simulink model "PR_Planar_Testbench_2018"  (R2024a)
settings: Solver=FixedStepDiscrete  StartTime=0.0  StopTime=inf  FixedStep=param.t_sample  RelTol=1e-3
undefined symbols (not defined in the file): max_qa, min_qa, param, slave3
libraries: Cust_Library_planarPKM x54, simulink_extras x27, dspswit3 x24, simulink x22, etherlab_lib x12
(part 1 of 6)
settings Model: SimulationMode=accelerator  ExtModeTrigDuration=10000  ExtModeArchiveMode=auto  ExtModeArchiveFileName=measurement_data  ExtModeArchiveDirName=/home/pkr_devpc/Schreibtisch/Git/3rrr_pkm/Versuchsstand/result  ExtModeLogAll=off  Creator=schappler  LastModifiedBy=mohammad_admin
settings SolverCC: AlgebraicLoopSolver=TrustRegion  MinimalZcImpactIntegration=on
settings DataIOCC: SaveOutput=off  SignalLogging=off  SaveTime=off  ReturnWorkspaceOutputs=off
settings OptimizationCC: BufferReuse=off  GlobalBufferReuse=off  ExpressionFolding=off  LocalBlockOutputs=off  OptimizeDataStoreBuffers=off  BusAssignmentInplaceUpdate=off
settings DebuggingCC: ReadBeforeWriteMsg=DisableAll  WriteAfterWriteMsg=DisableAll  WriteAfterReadMsg=DisableAll  MultiTaskDSMMsg=none  UnconnectedInputMsg=warning  UnconnectedOutputMsg=warning  UnconnectedLineMsg=warning  ArithmeticOperatorsInVariantConditions=warning
settings ModelReferenceCC: UpdateModelReferenceTargets=IfOutOfDate  EnableRefExpFcnMdlSchedulingChecks=on
settings SFSimCC: SFSimEcho=off  CustomCodeUndefinedFunction=UseInterfaceOnly
settings RTWCC: Description=EtherLab PREEMT_RT Real-Time Target  SystemTargetFile=etherlab.tlc  TemplateMakefile=etherlab_hrt.tmf  GenerateReport=on  LaunchReport=on  GPUComputeCapability=3.5
settings STFCustomTargetCC: UseToolchainInfoCompliant=off  SystemTargetFile=etherlab.tlc
settings GRTTargetCC: ParMdlRefBuildCompliant=off  CompOptLevelCompliant=off  ConcurrentExecutionCompliant=off  CombineOutputUpdateFcns=off  MatFileLogging=off  CPPClassGenCompliant=off  GRTInterface=on  UseToolchainInfoCompliant=off  ExtMode=on  ExtModeStaticAlloc=on  ExtModeStaticAllocSize=2000000000  ExtModeMexArgs='10.144.130.139' 0 17725  RTWCAPISignals=on  RTWCAPIParams=on

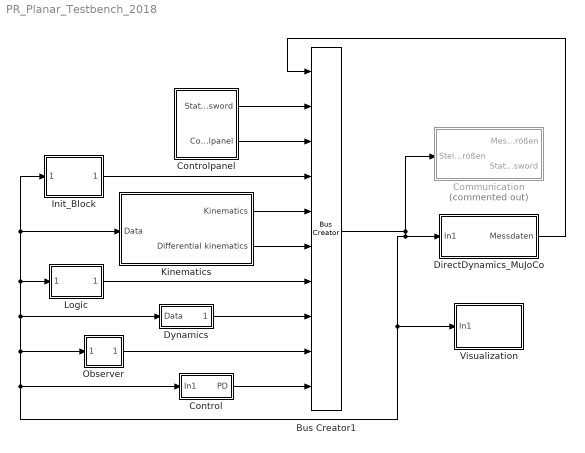
== system PR_Planar_Testbench_2018 ==
  Bus Creator1 : BusCreator  Inputs=10
  Communication : Subsystem  Commented=on
  Control : Subsystem
  Controlpanel : Subsystem
  DirectDynamics_MuJoCo : Subsystem
  Dynamics : Subsystem
  Init_Block : Subsystem
  Kinematics : Subsystem
  Logic : Subsystem
  Observer : Subsystem
  Visualization : Subsystem
  wires:
  Bus Creator1/1 -> Communication/1(Stellgrößen), Init_Block/1(Start_int), Kinematics/1(Data), Logic/1(Data), Dynamics/1(Data), Observer/1(In1), Control/1(In1), Visualization/1(In1), DirectDynamics_MuJoCo/1(In1)
  Control/1(PD) -> Bus Creator1/10
  Observer/1(Obs) -> Bus Creator1/9
  Dynamics/1(1) -> Bus Creator1/8
  Logic/1(Out1) -> Bus Creator1/7
  Kinematics/2(Differential kinematics) -> Bus Creator1/6
  Kinematics/1(Kinematics) -> Bus Creator1/5
  Init_Block/1(Out1) -> Bus Creator1/4
  Controlpanel/2(Controlpanel) -> Bus Creator1/3
  DirectDynamics_MuJoCo/1(Messdaten) -> Bus Creator1/1
  Controlpanel/1(Statusword) -> Bus Creator1/2

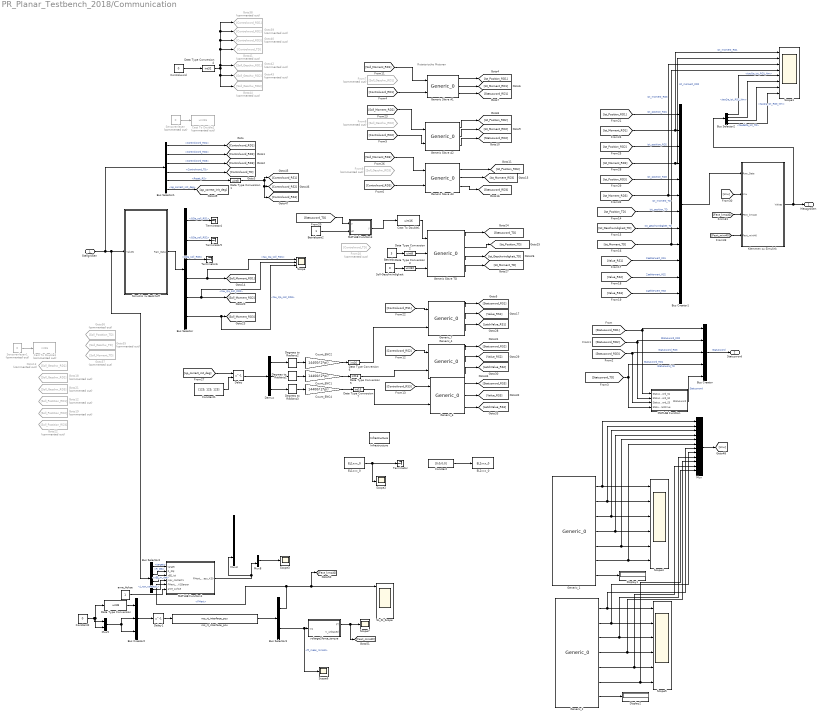
== system PR_Planar_Testbench_2018/Communication ==
  note: Rotatorische Motoren
  Stellgrößen : Inport
  Betriebsart : Constant  Value=3  SampleTime=-1
  Betriebsart2 : Constant  SampleTime=-1
  Bus Creator : BusCreator  Inputs=5
  Bus Creator1 : BusCreator  Inputs=12
  Bus Creator2 : BusCreator  Inputs=3
  Bus Selector : BusSelector  OutputSignals=QDa_soll_RD1,QDa_soll_RD2,QDa_soll_RD3,tau_Qa_soll_RD1,tau_Qa_soll_RD2,tau_Qa_soll_RD3
  Bus Selector1 : BusSelector  OutputSignals=State Variables.Controlword_RD1,State Variables.Controlword_RD2,State Variables.Controlword_RD3,State Variables.Controlword_TD,Controlpanel.Reset_RS,Kinematics_currentValues.qp_correct_init_deg
  Bus Selector2 : BusSelector  OutputSignals=tauQa_ist_RD1_Nm,tauQa_ist_RD2_Nm,tauQa_ist_RD3_Nm,taudelta_ist_TD
  Bus Selector3 : BusSelector  OutputSignals=FMext,ft_meas_mini40
  Bus Selector4 : BusSelector  OutputSignals=Controlpanel.target,Kontakt.R_0Gj,Kinematics_currentValues.xEE_m_rad,Kontakt.J_xpx_contact1
  Cast To Double1 : DataTypeConversion  OutDataTypeStr=uint16  SaturateOnIntegerOverflow=off  RndMeth=Floor
  Cast To Double2 : DataTypeConversion  Commented=on  OutDataTypeStr=uint16  SaturateOnIntegerOverflow=off  RndMeth=Floor
  Cast To Double3 : DataTypeConversion  Commented=on  OutDataTypeStr=int16  SaturateOnIntegerOverflow=off  RndMeth=Floor
  Constant : Constant  Value=[0;0;0;0]  SampleTime=param.t_sample
  Constant1 : Constant  Value=[123; 123; 123]  SampleTime=param.t_sample
  Constant2 : Constant  Value=0  SampleTime=-1
  "Controlword " : Constant  Value=0  SampleTime=-1
  Count_ENC1 : Gain  Gain=14400/(2*pi)  ParamDataTypeStr=double  OutDataTypeStr=double
  Count_ENC2 : Gain  Gain=14400/(2*pi)  ParamDataTypeStr=double  OutDataTypeStr=double
  Count_ENC4 : Gain  Gain=14400/(2*pi)  ParamDataTypeStr=double  OutDataTypeStr=double
  Data Type Conversion : DataTypeConversion  OutDataTypeStr=uint8  SaturateOnIntegerOverflow=off  RndMeth=Floor
  Data Type Conversion1 : DataTypeConversion  OutDataTypeStr=uint8  SaturateOnIntegerOverflow=off  RndMeth=Floor
  Data Type Conversion2 : DataTypeConversion  OutDataTypeStr=uint8  SaturateOnIntegerOverflow=off  RndMeth=Floor
  Data Type Conversion3 : DataTypeConversion  OutDataTypeStr=uint32  SaturateOnIntegerOverflow=off  RndMeth=Floor
  Data Type Conversion4 : DataTypeConversion  OutDataTypeStr=int32  SaturateOnIntegerOverflow=off  RndMeth=Floor
  Data Type Conversion5 : DataTypeConversion  OutDataTypeStr=int16  SaturateOnIntegerOverflow=off  RndMeth=Floor
  Data Type Conversion6 : DataTypeConversion  OutDataTypeStr=int16  SaturateOnIntegerOverflow=off  RndMeth=Floor
  Data Type Conversion7 : DataTypeConversion  OutDataTypeStr=int16  SaturateOnIntegerOverflow=off  RndMeth=Floor
  Degrees to Radians1 : simulink_extras/Transformations/Degrees to Radians
  Degrees to Radians2 : simulink_extras/Transformations/Degrees to Radians
  Degrees to Radians3 : simulink_extras/Transformations/Degrees to Radians
  Delay : Delay  DelayLength=1  InitialConditionSource=Input port  InitialCondition=[122;122;123]
      settings: InputPortMap=u0,p4
  Delay1 : Delay  DelayLength=1
  Demux : Demux  Outputs=3
  Display1 : Display
  Display2 : Display
  EL1xxx_0 : etherlab_lib/EtherCAT/Beckhoff/EL1xxx_0  master=0  index=6  model=EL1004  revision=[65810514 1048576]  vector=on  tsample=param.t_sample  debug=0
  EL2xxx_0 : etherlab_lib/EtherCAT/Beckhoff/EL2xxx_0  master=0  index=5  model=EL2004  revision=[131346514 1048576]  vector=on  diag=off  tsample=param.t_sample  debug=0
  From10 : From  Commented=on  GotoTag=Controlword_TD
  From7 : From  Commented=on  GotoTag=Soll_Geschw_RD1
  From8 : From  Commented=on  GotoTag=Soll_Geschw_RD2
  From9 : From  Commented=on  GotoTag=Soll_Geschw_RD3
  Generic Slave A1 : etherlab_lib/EtherCAT/Generic_0  master=0  index=1  rv=slave1_Stromregelung  param=[]  tsample=0.001  debug=0
  Generic Slave A2 : etherlab_lib/EtherCAT/Generic_0  master=0  index=2  rv=slave1_Stromregelung  param=[]  tsample=0.001  debug=0
  Generic Slave A3 : etherlab_lib/EtherCAT/Generic_0  master=0  index=0  rv=slave1_Stromregelung  param=[]  tsample=0.001  debug=0
  Generic Slave TD : etherlab_lib/EtherCAT/Generic_0  master=0  index=3  rv=slave3()  param=[]  tsample=0.001  debug=0
  Generic_1 : etherlab_lib/EtherCAT/Generic_0  master=0  index=10  rv=imu_etherlab_config  param=[]  tsample=1e-3  debug=0
  Generic_2 : etherlab_lib/EtherCAT/Generic_0  master=0  index=11  rv=imu_etherlab_config  param=[]  tsample=1e-3  debug=0
  Generic_4 : etherlab_lib/EtherCAT/Generic_0  master=0  index=9  rv=slave7  param=[]  tsample=0.001  debug=0
  Generic_6 : etherlab_lib/EtherCAT/Generic_0  master=0  index=7  rv=slave7  param=[]  tsample=0.001  debug=0
  Generic_7 : etherlab_lib/EtherCAT/Generic_0  master=0  index=8  rv=slave7  param=[]  tsample=0.001  debug=0
  Goto12 : Goto  Commented=on  GotoTag=Soll_Postition_RD1
  Goto13 : Goto  Commented=on  GotoTag=Soll_Geschw_RD1
  Goto18 : Goto  Commented=on  GotoTag=Soll_Geschw_RD2
  Goto19 : Goto  Commented=on  GotoTag=Soll_Postition_RD2
  Goto21 : Goto  Commented=on  GotoTag=Soll_Geschw_RD3
  Goto22 : Goto  Commented=on  GotoTag=Soll_Postition_RD3
  Goto35 : Goto  Commented=on  GotoTag=Soll_Geschw_TD
  Goto36 : Goto  Commented=on  GotoTag=Soll_Postition_TD
  Goto37 : Goto  Commented=on  GotoTag=Soll_Moment_TD
  Goto38 : Goto  Commented=on  GotoTag=Controlword_RD1
  Goto39 : Goto  Commented=on  GotoTag=Controlword_RD2
  Goto40 : Goto  Commented=on  GotoTag=Controlword_RD3
  Goto41 : Goto  Commented=on  GotoTag=Controlword_TD
  Goto42 : Goto  Commented=on  GotoTag=Soll_Geschw_RD1
  Goto43 : Goto  Commented=on  GotoTag=Soll_Geschw_RD2
  Goto44 : Goto  Commented=on  GotoTag=Soll_Geschw_RD3
  Infrastructure : etherlab_lib/EtherCAT/Beckhoff/Infrastructure  master=0  index=4  model=EK1100  revision=[72100946 0]  vector=off  tsample=param.t_sample  debug=0
  Klemmen zu Simulink : Subsystem
  MATLAB Function : MATLAB Function  TreatAsAtomicUnit=on
  MATLAB Function1 : MATLAB Function  TreatAsAtomicUnit=on
  MATLAB Function3 : MATLAB Function  TreatAsAtomicUnit=on
  Mux : Mux  Inputs=12
  Mux3 : Mux
  Mux5 : Mux  Inputs=2
  Mux8 : Mux  Inputs=2
  SL_IN_Scope : Scope  NumInputPorts=5
  Scope : Scope  NumInputPorts=3
  Scope1 : Scope  NumInputPorts=8
  Scope{2..3,6..7} (4 alike) : Scope
  Scope4 : Scope  NumInputPorts=6
  Scope5 : Scope  NumInputPorts=6
  Sensorenlesen : Constant  Commented=on  Value=0  SampleTime=-1
  Sensorenlesen1 : Constant  Commented=on  Value=0  SampleTime=-1
  Simulink zu Beckhoff : Subsystem
  Soll-Geschwindigkeit : Constant  Value=0  SampleTime=-1
  Terminator{,4..6} (4 alike) : Terminator
  anre_Achse : Constant  SampleTime=-1
  ros_rt_interface_pcu : S-Function  FunctionName=ros_rt_interface_pcu  SFunctionDeploymentMode=off  EnableBusSupport=off  mask(Legacy Function){SFunctionSpec=void SL_io_func(SL_OUT_type u1[1], SL_IN_type y1[1]), ShowSpec=on}
      mask prompts: ShowSpec "Display function specification"
      mask help:
      | This block allows you to call the legacy functions specified by the following Legacy Code Tool definition:
      | def.SFunctionName = 'ros_rt_interface_pcu';
      | def.OutputFcnSpec = 'void SL_io_func(SL_OUT_type u1[1], SL_IN_type y1[1])';
      | def.StartFcnSpec = 'void SL_start_func()';
      | def.TerminateFcnSpec = 'void SL_terminate_func()';
      | def.HeaderFiles = {'SL_func.h'};
      | def.SourceFiles = {'../ros_rt_interface/ros_rt_core/SL_func_dummy.cpp'};
      | def.TargetLibFiles = {'libros_sl_interface.so'};
      | def.IncPaths = {'../ros_rt_interface/ros_rt_core'};
      mask Help: <p>This block was generated automatically by the Legacy Code Tool. For detailed help on this tool, call<a href="matlab:legacy_code('help')"> legacy_code('help')</a>.</p>
      mask Callback ShowSpec:
      | if strcmp(get_param(gcbh, 'ShowSpec'), 'on')
      |   set_param(gcbh, 'MaskDisplay', sprintf('fprintf(''%s'');', get_param(gcbh, 'SFunctionSpec')));
      | else
      |   set_param(gcbh, 'MaskDisplay', sprintf('fprintf(''%s'');', get_param(gcbh, 'FunctionName')));
      | end
      mask Display: fprintf('void SL_io_func(SL_OUT_type u1[1], SL_IN_type y1[1])');
  voltage2force_torque : Subsystem
  Messgrößen : Outport
  Statusword : Outport  Port=2
  wires:
  [Ist_Moment_RD2] -> Scope1/2, Bus Creator1/4  "ist_moment_RD2"
  [Ist_Position_RD2] -> Bus Creator1/3  "Ist_position_RD2"
  Klemmen zu Simulink/1(Values) -> Bus Selector2/1, Messgrößen/1
  [Ist_Moment_RD3] -> Bus Creator1/6, Scope1/3  "ist_moment_RD3"
  [Ist_Position_RD1] -> Bus Creator1/1  "Ist_position_RD1"
  [Ist_Moment_RD1] -> Scope1/1, Bus Creator1/2  "ist_moment_RD1"
  Bus Creator1/1 -> Klemmen zu Simulink/1(Raw_Data)
  [Ist_Position_RD3] -> Bus Creator1/5  "Ist_position_RD3"
  Simulink zu Beckhoff/1(Raw_Data) -> Bus Selector/1
  [Statusword_RD2] -> MATLAB Function/2(Statusword_S2), Bus Creator/2  "Statusword_RD2"
  [Statusword_RD3] -> MATLAB Function/3(Statusword_S3), Bus Creator/3  "Statusword_RD3"
  [Statusword_RD1] -> MATLAB Function/1(Statusword_S1), Bus Creator/1  "Statusword_RD1"
  MATLAB Function/1(Statusword) -> Bus Creator/5  "Statusword"
  Bus Creator/1 -> Statusword/1  "Statusword"
  [Statusword_TD] -> Bus Creator/4, MATLAB Function/4(Statusword_TranslDrive)  "Statusword_TD"
  [Controlword_RD2] -> Generic Slave A2/2
  [Controlword_RD3] -> Generic Slave A3/2
  [Controlword_RD1] -> Generic Slave A1/2
  Betriebsart/1 -> Data Type Conversion2/1
  Generic Slave A1/2 -> [Ist_Moment_RD1]
  Generic Slave A1/3 -> [Statusword_RD1]
  Generic Slave A2/1 -> [Ist_Position_RD2]
  Generic Slave A2/2 -> [Ist_Moment_RD2]
  Generic Slave A2/3 -> [Statusword_RD2]
  Generic Slave A3/1 -> [Ist_Position_RD3]
  Generic Slave A3/2 -> [Ist_Moment_RD3]
  Generic Slave A3/3 -> [Statusword_RD3]
  Generic Slave TD/1 -> [Statusword_TD]
  Generic Slave TD/2 -> [Ist_Position_TD]
  Generic Slave TD/3 -> [Ist_Geschwindigkeit_TD]
  Generic Slave TD/4 -> [Ist_Moment_TD]
  Soll-Geschwindigkeit/1 -> Data Type Conversion3/1
  Data Type Conversion6/1 -> Generic_7/2
  Generic_7/3 -> [LatchValue_RS1]
  Generic_7/2 -> [Value_RS1]
  Generic_7/1 -> [Statusword_RS1]
  Generic_6/2 -> [Value_RS3]
  Generic_6/3 -> [LatchValue_RS3]
  Generic_6/1 -> [Statusword_RS3]
  Generic_4/3 -> [LatchValue_RS2]
  Generic_4/2 -> [Value_RS2]
  Generic_4/1 -> [Statusword_RS2]
  [Ist_Position_TD] -> Bus Creator1/7  "Ist_position_TD"
  [Ist_Geschwindigkeit_TD] -> Bus Creator1/8  "Ist_geschwindigkeit_TD"
  [Ist_Moment_TD] -> Scope1/4, Bus Creator1/9  "Ist_moment_TD"
  [Value_RS1] -> Bus Creator1/10  "Zaehlerwert_RS1"
  [Value_RS2] -> Bus Creator1/11  "Zaehlerwert_RS2"
  [Value_RS3] -> Bus Creator1/12  "Zaehlerwert_RS3"
  "Controlword "/1 -> Data Type Conversion4/1
  Generic Slave A1/1 -> [Ist_Position_RD1]
  Bus Selector1/5 -> Data Type Conversion1/1  "<Reset_RS>"
  [Controlword_RS2] -> Generic_4/1
  [Controlword_RS3] -> Generic_6/1
  Data Type Conversion1/1 -> [Controlword_RS3], [Controlword_RS2], [Controlword_RS1]
  [Controlword_RS1] -> Generic_7/1
  Data Type Conversion2/1 -> Generic Slave TD/2
  Data Type Conversion3/1 -> Generic Slave TD/3
  Data Type Conversion4/1 -> Goto38/1, Goto39/1, Goto40/1, Goto41/1, Goto42/1, Goto44/1, Goto43/1
  Betriebsart2/1 -> MATLAB Function3/2(u2)
  [Statusword_TD] -> MATLAB Function3/1(u)
  MATLAB Function3/1(y) -> Cast To Double1/1
  Bus Selector/4 -> [Soll_Moment_RD1], Scope/1  "<tau_Qa_soll_RD1>"
  Bus Selector/5 -> Scope/2, [Soll_Moment_RD2]  "<tau_Qa_soll_RD2>"
  Bus Selector/6 -> Scope/3, [Soll_Moment_RD3]  "<tau_Qa_soll_RD3>"
  [Soll_Moment_RD1] -> Generic Slave A1/1
  [Soll_Moment_RD2] -> Generic Slave A2/1
  [Soll_Moment_RD3] -> Generic Slave A3/1
  Bus Selector2/1 -> Scope1/5  "<tauQa_ist_RD1_Nm>"
  Bus Selector2/2 -> Scope1/6  "<tauQa_ist_RD2_Nm>"
  Bus Selector2/3 -> Scope1/7  "<tauQa_ist_RD3_Nm>"
  Bus Selector2/4 -> Scope1/8  "<taudelta_ist_TD>"
  Cast To Double1/1 -> Generic Slave TD/1
  Bus Selector1/1 -> [Controlword_RD1]  "<Controlword_RD1>"
  Bus Selector1/2 -> [Controlword_RD2]  "<Controlword_RD2>"
  Bus Selector1/4 -> [Controlword_TD]  "<Controlword_TD>"
  Bus Selector1/3 -> [Controlword_RD3]  "<Controlword_RD3>"
  Bus Selector/1 -> Terminator4/1  "<QDa_soll_RD1>"
  Bus Selector/2 -> Terminator5/1  "<QDa_soll_RD2>"
  Bus Selector/3 -> Terminator6/1  "<QDa_soll_RD3>"
  Sensorenlesen/1 -> Cast To Double2/1
  Sensorenlesen1/1 -> Cast To Double3/1
  EL1xxx_0/1 -> Scope2/1, Terminator/1
  Constant/1 -> EL2xxx_0/1
  Bus Selector1/6 -> [qp_correct_init_deg]  "<qp_correct_init_deg>"
  Count_ENC2/1 -> Data Type Conversion6/1
  [qp_correct_init_deg] -> Delay/1
  Count_ENC4/1 -> Data Type Conversion7/1
  Demux/1 -> Degrees to Radians2/1
  Demux/2 -> Degrees to Radians1/1
  Constant1/1 -> Delay/2
  Degrees to Radians1/1 -> Count_ENC1/1
  Count_ENC1/1 -> Data Type Conversion5/1
  Delay/1 -> Demux/1
  Degrees to Radians2/1 -> Count_ENC2/1
  Degrees to Radians3/1 -> Count_ENC4/1
  Demux/3 -> Degrees to Radians3/1
  Data Type Conversion5/1 -> Generic_4/2
  Data Type Conversion7/1 -> Generic_6/2
  Generic_1/6 -> Mux/6, Scope4/6
  Generic_2/3 -> Scope5/3, Mux/9
  Generic_2/1 -> Scope5/1, Mux/7
  Mux/1 -> [imu]
  Generic_1/3 -> Scope4/3, Mux/3
  Generic_1/4 -> Scope4/4, Mux/4
  Generic_1/7 -> Display1/1
  Generic_2/7 -> Display2/1
  Generic_1/5 -> Mux/5, Scope4/5
  Generic_2/4 -> Scope5/4, Mux/10
  Generic_2/2 -> Scope5/2, Mux/8
  Generic_1/1 -> Scope4/1, Mux/1
  Generic_1/2 -> Scope4/2, Mux/2
  Generic_2/6 -> Scope5/6, Mux/12
  Generic_2/5 -> Scope5/5, Mux/11
  [imu] -> Klemmen zu Simulink/2(imu)
  Bus Selector4/3 -> MATLAB Function1/3(xEE_ist)  "<xEE_m_rad>"
  Constant2/1 -> Mux5/2, Data Type Conversion/1, Mux5/1
  Delay1/1 -> ros_rt_interface_pcu/1
  Mux8/1 -> Scope3/1
  Bus Selector4/1 -> MATLAB Function1/1(target)  "<target>"
  Bus Selector4/2 -> MATLAB Function1/2(R_0Gj)  "<R_0Gj>"
  ros_rt_interface_pcu/1 -> Bus Selector3/1
  MATLAB Function1/1(FMext_mobPlat_mess_KS0) -> Mux8/2, Mux3/4
  voltage2force_torque/1(FT) -> [Fext_mini40], Scope7/1
  Bus Selector3/1 -> MATLAB Function1/5(FMext_link_KSSensor), [Fext_kms40], SL_IN_Scope/1  "<FMext>"
  Mux5/1 -> Bus Creator2/3, Bus Creator2/2
  Bus Creator2/1 -> Delay1/1
  Bus Selector3/2 -> Scope6/1, voltage2force_torque/1(In1)  "<ft_meas_mini40>"
  Stellgrößen/1 -> Bus Selector1/1, Bus Selector4/1, Simulink zu Beckhoff/1(Values)
  Bus Selector4/4 -> MATLAB Function1/4(Jxpx_contact1)  "<J_xpx_contact1>"
  Data Type Conversion/1 -> Bus Creator2/1
  anre_Achse/1 -> MATLAB Function1/6(anre_Achse)
  [Fext_kms40] -> Klemmen zu Simulink/3(Fext_kms40)
  [Fext_mini40] -> Klemmen zu Simulink/4(Fext_mini40)

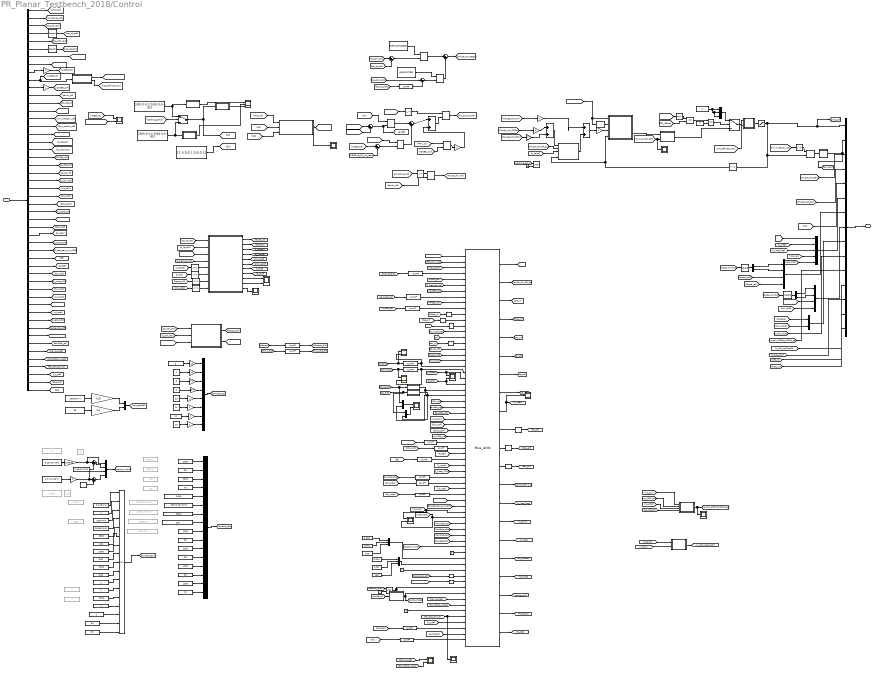
== system PR_Planar_Testbench_2018/Control ==
  note: Redundanzauflösung mit Task-Prio auf Geschwindigkeitsebene
  note: Berechnung der Steifigkeits- und Dämpfungsparameter für den kartesischen Impedanzregler
  note: Momentenvorsteuerung der Zentrifugaleffekte für Impedanzgesetz des geschl. Regelkreises
  note: Impedanzregler mit Momentenvorsteuerung der Dynamikeffekte (Trägheit und Zentrifugal) für Impedanzgesetz des geschl. Regelkreises
  note: PD-Regler im Gelenkraum
  In1 : Inport
  AND1 : Logic  Operator=OR  AllPortsSameDT=off  OutDataTypeStr=boolean
  Bus Creator1 : BusCreator  Inputs=15
  Bus Selector : BusSelector  OutputSignals=Dynamik.MMX,Differential kinematics - current values.J_hredxqa,Logical data.Qa_des_rad,Kinematics_currentValues.Qa_rad_m,Logical data.QDa_des_rads,Differential kinematics - current values.QDa_rads_ms,Logical data.xEE_des_m_rad,Kinematics_currentValues.xEE_m_rad,Logical data.xDEE_des_ms_rads,Differential kinematics - current values.xDEE_ms_rads,Logical data.xDDEE_des_mss_radss,Dynamik.taucX,Logical data.BP_isError,Controlpanel.Enable_Drive,Differential kinematics - current values.Jinv_hredqax,Logical data.turn_control_off,Logical data.retraction_active,Kinematics_currentValues.Q_rad,Differential kinematics - current values.dJ_hredxqa,Dynamik.MMQa,Dynamik.taucQa,Beobachter.alpha_nf,Logical data.Q_des_rad,Logical data.xp_des,Logical data.dxp_des,Logical data.ddxp_des,Beobachter.xp_KSGj,Beobachter.dxp_KSGj,Beobachter.dRxp,Beobachter.J_xpqa,Beobachter.J_xpqa_KS0,Logical data.BP_Retr_calc_run_xp,Beobachter.dR,Beobachter.R_0Gj,Beobachter.dJ_xpqa,Beobachter.dJ_xpqa_KS0,Beobachter.dxp_KS0,Beobachter.xp_KS0,Beobachter.predbody_sel,Controlpanel.rr_level,Controlpanel.retr_CS0,Logical data.kappa_traj_des,Logical data.mindist_traj_des,Dynamik.Cred_Qa,Beobachter.clamping_predicted,Beobachter.clampingChain_predicted,Logical data.traj_qap_soll_cl,Differential kinematics - current values.Jinv_hqx_dq_dqa,Differential kinematics - current values.dJinv_hqx_dq_dqa,Differential kinematics - current values.QD_mod_rads
  Constant1 : Constant  SampleTime=-1
  Constant13 : Constant  Value=10000*0.4  SampleTime=-1
  Constant14 : Constant  SampleTime=-1
  Constant16 : Constant  Value=85  SampleTime=-1
  Constant2 : Constant  SampleTime=-1
  Constant3 : Constant  Value=0  SampleTime=-1
  Constant7 : Constant  Value=eye(3,3)*10000  SampleTime=-1
  Constant8 : Constant  Value=eye(3,3)*85  SampleTime=-1
  Dd : Constant  Value=[1 0 0;0 1 0;0 0 1]  SampleTime=-1
  Delay{,1..2,8} (4 alike) : Delay  DelayLength=1  InitialCondition=zeros(3,1)
  Delay13 : Delay  DelayLength=1  InitialCondition=[9 0 0]
  Delay14 : Delay  DelayLength=1  InitialCondition=[0.175 0 0]
  Delay3 : Delay  DelayLength=1  InitialCondition=zeros(1,3)
  Delay4 : Delay  DelayLength=1  InitialCondition=zeros(1,3)
  Delay5 : Delay  DelayLength=1  InitialCondition=8
  Delay6 : Delay  DelayLength=1  InitialCondition=0.17
  Delay7 : Delay  DelayLength=1  InitialCondition=1
  Demux4 : Demux  Outputs=2
  Demux5 : Demux  Outputs=2
  Edge Detector : dspswit3/Edge Detector  InputProcessing=Columns as channels (frame based)
  Equal : RelationalOperator  Operator===  OutDataTypeStr=boolean  RndMeth=Simplest  InputSameDT=off
  Gain{,1..2,4,6,12..14,17} (9 alike) : Gain
  Gain10 : Gain  Gain=0
  Gain11 : Gain  Gain=3*2
  Gain15 : Gain  Gain=0.25
  Gain16 : Gain  Gain=0.4
  Gain3 : Gain  Gain=10
  Gain5 : Gain  Gain=10
  Gain7 : Gain  Gain=0
  Gain8 : Gain  Gain=2*2
  Kd : Constant  Value=[2000 0 0;0 2000 0;0 0 85]  SampleTime=-1
  Kd_react : Constant  Value=[2000 0 0;0 2000 0;0 0 85]  SampleTime=-1
  Logical Operator : Logic  AllPortsSameDT=off  OutDataTypeStr=boolean
  Logical Operator1 : Logic  AllPortsSameDT=off  OutDataTypeStr=boolean
  LowPF{,2..3,11} (4 alike) : Cust_Library_planarPKM/LowPF  f_lp=param.f_lp_Hz  t_sample=param.t_sample  initial_value=zeros(3,3)
  LowPF1 : Cust_Library_planarPKM/LowPF  f_lp=param.f_lp_Hz  t_sample=param.t_sample  initial_value=[0;0;0]
  LowPF{5,10,12..13} (4 alike) : Cust_Library_planarPKM/LowPF  f_lp=param.f_lp_Hz  t_sample=param.t_sample  initial_value=zeros(3,1)
  LowPF16 : Cust_Library_planarPKM/LowPF  f_lp=param.f_lp_Hz  t_sample=param.t_sample  initial_value=zeros(9,1)
  LowPF17 : Cust_Library_planarPKM/LowPF  f_lp=param.f_lp_Hz  t_sample=param.t_sample  initial_value=zeros(9,3)
  LowPF{8..9,18..19} (4 alike) : Cust_Library_planarPKM/LowPF  f_lp=param.f_lp_Hz  t_sample=param.t_sample  initial_value=zeros(1,1)
  LowPF4 : Cust_Library_planarPKM/LowPF  f_lp=param.f_lp_Hz  t_sample=param.t_sample  initial_value=zeros(2,1)
  MATLAB Function : MATLAB Function  TreatAsAtomicUnit=on
  MATLAB Function1 : MATLAB Function  TreatAsAtomicUnit=on
  MATLAB Function10 : MATLAB Function  TreatAsAtomicUnit=on
  MATLAB Function12 : MATLAB Function  TreatAsAtomicUnit=on
  MATLAB Function13 : MATLAB Function  TreatAsAtomicUnit=on
  MATLAB Function2 : MATLAB Function  TreatAsAtomicUnit=on
  MATLAB Function3 : MATLAB Function  TreatAsAtomicUnit=on
  MATLAB Function4 : MATLAB Function  TreatAsAtomicUnit=on
  MATLAB Function5 : MATLAB Function  TreatAsAtomicUnit=on
  MATLAB Function6 : MATLAB Function  TreatAsAtomicUnit=on
  MATLAB Function7 : MATLAB Function  TreatAsAtomicUnit=on
  MATLAB Function8 : MATLAB Function  TreatAsAtomicUnit=on
  MATLAB Function9 : MATLAB Function  TreatAsAtomicUnit=on
  Matrix Multiply : Product  Multiplication=Matrix(*)
  MatrixMultiply{1..2,4..6,8,11} (7 alike) : Product  Multiplication=Matrix(*)
  Moe_ArMo : Cust_Library_planarPKM/Moe_ArMo  SystemSampleTime=-1  VariantActivationTime=update diagram  AllowFlexibleInterface=on  Latency=0  AutoFrameSizeCalculation=off
  Mux : Mux  Inputs=3
  Mux21 : Mux  Inputs=16
  Mux22 : Mux  Inputs=17
  Mux{23..24,31..32} (4 alike) : Mux  Inputs=2
  Mux25 : Mux  Inputs=5
  Mux26 : Mux
  Mux27 : Mux
  Mux28 : Mux
  Mux36 : Mux  Inputs=3
  Mux37 : Mux  Inputs=3
  Mux5 : Mux  Inputs=8
  NOT5 : Logic  Operator=NOT  AllPortsSameDT=off  OutDataTypeStr=boolean
  PD_Saturation_X : Saturate  UpperLimit=50  LowerLimit=-50
  Reshape : Reshape
  Reshape2 : Reshape
  Reshape4 : Reshape
  Scope{7,12,14..15,22..23,26..27} (8 alike) : Scope  NumInputPorts=2
  Scope{2,4..5,9,29..30} (6 alike) : Scope
  Scope6 : Scope  NumInputPorts=3
  Selector : Selector  InputPortWidth=4  IndexOptions=Index vector (dialog)  Indices=[1 2 3]  OutputSizes=1
  Selector1 : Selector  InputPortWidth=4  IndexOptions=Index vector (dialog)  Indices=[1 2 3]  OutputSizes=1
  Selector6 : Selector  InputPortWidth=4  IndexOptions=Index vector (dialog)  Indices=[1 2]  OutputSizes=1
  Selector7 : Selector  InputPortWidth=4  IndexOptions=Index vector (dialog)  Indices=[3 4]  OutputSizes=1
  Sum{,2,6..7,9..10} (6 alike) : Sum  Inputs=|++
  Sum{1,3..5,8} (5 alike) : Sum  Inputs=|+-
  Switch : Switch  Criteria=u2 > Threshold  SaturateOnIntegerOverflow=off  InputSameDT=off
  Switch3 : Switch  Criteria=u2 > Threshold  SaturateOnIntegerOverflow=off  InputSameDT=off
  TP1_impl : Subsystem
  TP1_impl10 : Subsystem
  TP1_impl9 : Subsystem
  Transpose1 : Math  Operator=transpose  SignedPower=on
  Transpose2 : Math  Operator=transpose  SignedPower=on
  Transpose3 : Math  Operator=transpose  SignedPower=on
  Triggered Subsystem : Subsystem  TreatAsAtomicUnit=on
  activate_bp_UNB : Constant  Value=0  SampleTime=-1
  clampingreaction_active : Constant  Value=0  SampleTime=-1
  const : Constant  Value=0.25+1.75*0  SampleTime=-1
  const1 : Constant  Value=0.005  SampleTime=-1
  const2 : Constant  Commented=on  Value=0.02  SampleTime=-1
  const3 : Constant  Commented=on  Value=10  SampleTime=-1
  decimal_point_zero : Constant  Value=0.001  SampleTime=-1
  decimal_point_zero1 : Constant  Value=0.001  SampleTime=-1
  kappa_gain : Gain  Gain=100000
  kappa_lim : Constant  Value=9.25+23.75*0  SampleTime=-1
  kappa_lim1 : Constant  Commented=on  Value=9  SampleTime=-1
  lambda_clamp_dqa_tau : Constant  Value=35  SampleTime=-1
  lambda_clamp_dqap_ddqa : Constant  Value=75  SampleTime=-1
  lambda_clamp_dqap_tau_enkoppeln : Constant  Value=0  SampleTime=-1
  lambda_clamp_dqp_tau : Constant  Value=30  SampleTime=-1
  lambda_clamp_qap : Constant  Value=10  SampleTime=-1
  lambda_clamp_qap_ddqa : Constant  Value=1250  SampleTime=-1
  lambda_clamp_qap_tau : Constant  Value=1000  SampleTime=-1
  lambda_clamp_qap_tau_entkoppelt : Constant  SampleTime=-1
  lambda_ddist_ddqa : Constant  Value=100  SampleTime=-1
  lambda_ddist_ddqa1 : Constant  Commented=on  Value=500*0.5  SampleTime=-1
  lambda_ddist_tau : Constant  Value=20000*0.01  SampleTime=-1
  lambda_dist : Constant  Value=5  SampleTime=-1
  lambda_dist_ddqa : Constant  Value=1500  SampleTime=-1
  lambda_dist_ddqa1 : Constant  Commented=on  Value=1250*0.5  SampleTime=-1
  lambda_dist_tau : Constant  Value=2000*4*2  SampleTime=-1
  lambda_dist_tau1 : Constant  Commented=on  Value=2000  SampleTime=-1
  lambda_dkappa_ddqa : Constant  Value=250*0.25*0.5*2  SampleTime=-1
  lambda_dkappa_ddqa1 : Constant  Commented=on  Value=250*0.25*0.5  SampleTime=-1
  lambda_dkappa_tau : Constant  SampleTime=-1
  lambda_dkappa_tau_entkoppelt : Constant  Value=2  SampleTime=-1
  lambda_dkappa_tau_entkoppelt1 : Constant  Commented=on  Value=4  SampleTime=-1
  lambda_dmindist_tau_entkoppelt : Constant  Value=2  SampleTime=-1
  lambda_dmindist_tau_entkoppelt1 : Constant  Commented=on  Value=4  SampleTime=-1
  lambda_dposxy_ddqa : Constant  Value=50  SampleTime=-1
  lambda_dposxy_ddqa1 : Constant  Commented=on  Value=100*0.5  SampleTime=-1
  lambda_dxp_ddqa : Constant  Value=50  SampleTime=-1
  lambda_dxp_qa_ddqa : Constant  Value=50  SampleTime=-1
  lambda_dxp_qa_tau : Constant  Value=100  SampleTime=-1
  lambda_dxp_tau : Constant  Value=300  SampleTime=-1
  lambda_dxpy_ddqa : Constant  Value=50  SampleTime=-1
  lambda_dxpy_tau : Constant  Value=300  SampleTime=-1
  lambda_dz_ddqa : Constant  Value=75  SampleTime=-1
  lambda_dz_ddqa1 : Constant  Commented=on  Value=75  SampleTime=-1
  lambda_kappa : Constant  Value=5  SampleTime=-1
  lambda_kappa_ddqa : Constant  Value=1500  SampleTime=-1
  lambda_kappa_ddqa1 : Constant  Commented=on  Value=1000*0.25*0.5  SampleTime=-1
  lambda_kappa_tau : Constant  Value=0.125*4*2  SampleTime=-1
  lambda_kappa_tau1 : Constant  Commented=on  Value=0.125  SampleTime=-1
  lambda_posxy : Constant  Value=3  SampleTime=-1
  lambda_posxy_ddqa : Constant  Value=2000  SampleTime=-1
  lambda_posxy_ddqa1 : Constant  Commented=on  Value=800*0.7  SampleTime=-1
  lambda_xp : Constant  Value=10  SampleTime=-1
  lambda_xp_ddqa : Constant  Value=1250  SampleTime=-1
  lambda_xp_qa : Constant  Value=10  SampleTime=-1
  lambda_xp_qa_ddqa : Constant  Value=1250  SampleTime=-1
  lambda_xp_qa_tau : Constant  Value=2500  SampleTime=-1
  lambda_xp_tau : Constant  Value=2000  SampleTime=-1
  lambda_xpy : Constant  Value=10  SampleTime=-1
  lambda_xpy_ddqa : Constant  Value=1000  SampleTime=-1
  lambda_xpy_tau : Constant  Value=2000  SampleTime=-1
  lambda_z : Constant  Value=4  SampleTime=-1
  lambda_z_ddqa : Constant  Value=2500  SampleTime=-1
  lambda_z_ddqa1 : Constant  Commented=on  Value=400  SampleTime=-1
  mindist_gain : Gain  Gain=0
  mindist_lim_m : Constant  Value=0.17-0.145*0  SampleTime=-1
  mindist_lim_m1 : Constant  Commented=on  Value=0.155  SampleTime=-1
  priority_x : Constant  Value=0  SampleTime=-1
  round_decimal_point_zero : Constant  Value=1e3  SampleTime=-1
  round_decimal_point_zero1 : Constant  Value=1e3  SampleTime=-1
  status_lbound : Constant  Value=0.001  SampleTime=-1
  status_lbound1 : Constant  Value=0.001  SampleTime=-1
  PD : Outport
  wires:
  In1/1 -> Bus Selector/1
  Bus Selector/1 -> [MMX_ist]  "<MMX>"
  Kd/1 -> Switch/3, MATLAB Function4/1(u)
  [Kd] -> MATLAB Function3/2(K_d)
  MATLAB Function3/1(D_d) -> Scope4/1, [Dd_unshaped]
  Dd/1 -> [Dd]
  Constant7/1 -> MatrixMultiply1/1
  PD_Saturation_X/1 -> Bus Creator1/1, [tauQ_soll], Delay/1, Matrix Multiply/2  "TauQa_soll_PD"
  Bus Creator1/1 -> PD/1  "PD_Controller"
  Bus Selector/2 -> [J_hredxqa_ist]  "<J_hredxqa>"
  Sum1/1 -> MatrixMultiply1/2
  Sum3/1 -> MatrixMultiply2/2  "de_Qa"
  Bus Selector/4 -> Selector/1  "<Qa_rad_m>"
  Bus Selector/3 -> [qa_soll_rad]  "<Qa_des_rad>"
  Selector/1 -> [qa_ist_rad]
  Bus Selector/5 -> [dqa_soll_rads]  "<QDa_des_rads>"
  Bus Selector/6 -> Selector1/1  "<QDa_rads_ms>"
  Transpose1/1 -> MatrixMultiply11/1
  [J_hredxqa_ist] -> Transpose1/1
  Constant2/1 -> Equal/2
  Equal/1 -> Switch3/2
  Mux/1 -> Switch3/1
  Switch3/1 -> MATLAB Function/1(u)
  Bus Selector/13 -> [BP_isError]  "<BP_isError>"
  Bus Selector/15 -> [Jinv_hredqax_ist]  "<Jinv_hredqax>"
  [Jinv_hredqax_ist] -> Transpose3/1
  Matrix Multiply/1 -> MATLAB Function1/1(u)
  Transpose3/1 -> Matrix Multiply/1
  MatrixMultiply1/1 -> Sum/1  "P"
  Bus Selector/14 -> [Enable_Drive]  "<Enable_Drive>"
  [BP_isError] -> AND1/2
  [Enable_Drive] -> NOT5/1
  NOT5/1 -> AND1/1
  AND1/1 -> Equal/1
  Constant3/1 -> Mux/3, Mux/2, Mux/1
  MatrixMultiply2/1 -> Sum/2  "D"
  Selector1/1 -> [dqa_ist_rads]
  MATLAB Function/1(y) -> PD_Saturation_X/1
  MATLAB Function1/1(y) -> [tauX_soll], Bus Creator1/2  "tauX_soll_PD"
  Bus Selector/16 -> [turn_control_off]  "<turn_control_off>"
  [turn_control_off] -> Scope2/1, MATLAB Function2/2(turn_control_off)
  Bus Selector/7 -> [xEE_soll_m_rad]  "<xEE_des_m_rad>"
  Bus Selector/8 -> [xEE_ist_m_rad]  "<xEE_m_rad>"
  Bus Selector/10 -> [xDEE_ist], TP1_impl/1(u_raw)  "<xDEE_ms_rads>"
  Bus Selector/11 -> Gain1/1  "<xDDEE_des_mss_radss>"
  Bus Selector/12 -> [taucX_ist]  "<taucX>"
  [dqa_ist_rads] -> LowPF13/1  "de_Qa"
  Constant8/1 -> MatrixMultiply2/1
  [taucX_ist] -> MatrixMultiply11/2
  [MMX_ist] -> MATLAB Function3/1(M)
  TP1_impl/1(u_filt) -> [xDEE_ist_filt_ms_rads]
  Bus Selector/9 -> Gain/1  "<xDEE_des_ms_rads>"
  Sum4/1 -> MatrixMultiply4/2, [exEE]
  [Kd] -> MatrixMultiply4/1
  [Dd_unshaped] -> MatrixMultiply5/1
  MatrixMultiply5/1 -> Sum6/2  "D"
  Sum5/1 -> MatrixMultiply5/2
  MatrixMultiply4/1 -> Sum6/1  "P"
  [J_hredxqa_ist] -> Transpose2/1
  Transpose2/1 -> MatrixMultiply8/1
  TP1_impl/2(not_defined_nan) -> [not_defined_nan]
  [not_defined_nan] -> MATLAB Function/2(not_defined_nan)
  [Kd] -> Bus Creator1/5  "Kd_xyphie"
  [Dd] -> MATLAB Function3/3(D)
  Gain1/1 -> [xDDEE_soll]
  Gain/1 -> [xDEE_soll]
  Bus Selector/17 -> [rueckzug_aktiv]  "<retraction_active>"
  [rueckzug_aktiv] -> Switch/2
  Switch/1 -> MATLAB Function6/1(u), [Kd]
  Kd_react/1 -> MATLAB Function5/1(u), Switch/1
  MATLAB Function5/1(y) -> Scope6/1
  MATLAB Function4/1(y) -> Scope6/2
  MATLAB Function6/1(y) -> Scope6/3
  Bus Selector/18 -> [q_ist_rad]  "<Q_rad>"
  [qa_ist_rad] -> Sum1/2
  [qa_soll_rad] -> Sum1/1
  [dqa_soll_rads] -> Sum3/1
  [xEE_ist_m_rad] -> Sum4/2
  [xEE_soll_m_rad] -> Sum4/1
  [xDEE_soll] -> Sum5/1
  [xDEE_ist_filt_ms_rads] -> Sum5/2
  Sum/1 -> [TauQa_Nm_PDQa]
  MatrixMultiply11/1 -> [TauQa_Nm_MV]
  [TauQa_Nm_MV] -> Gain10/1
  [TauQa_Nm_PDX] -> Gain4/1
  [TauQa_Nm_PDQa] -> Gain7/1
  [TauQa_Nm_MV] -> Bus Creator1/4  "TauQa_Nm_MV"
  [TauQa_Nm_PDX] -> Bus Creator1/3  "TauQa_Nm_PDX"
  [xEE_ist_m_rad] -> Moe_ArMo/2
  [qa_ist_rad] -> Moe_ArMo/3
  [J_hredxqa_ist] -> Moe_ArMo/6
  Moe_ArMo/1 -> [mode]  "mode"
  Moe_ArMo/2 -> [TauQa_Nm_RR_dq]
  [xDEE_soll] -> Moe_ArMo/5
  [xEE_soll_m_rad] -> Moe_ArMo/1
  [xDDEE_soll] -> Moe_ArMo/7
  Bus Selector/19 -> [dJ_hredxqa]  "<dJ_hredxqa>"
  Bus Selector/20 -> [MMQa_ist]  "<MMQa>"
  [MMQa_ist] -> Moe_ArMo/9
  Moe_ArMo/4 -> [ddqa_rr]
  Delay/1 -> MATLAB Function9/4(tau_prev), MATLAB Function7/5(tau_prev)
  Moe_ArMo/8 -> [qa_soll]
  MATLAB Function2/1(y) -> Switch3/3
  Delay1/1 -> Moe_ArMo/11
  [ddqa_rr] -> Delay1/1
  MATLAB Function7/1(tau_out) -> Sum2/2
  [dqa_rr] -> Delay2/1
  Delay2/1 -> Moe_ArMo/12
  Moe_ArMo/9 -> Scope5/1, [h_inter]
  Moe_ArMo/10 -> Reshape/1
  Moe_ArMo/7 -> [de_qa]
  Moe_ArMo/6 -> [e_qa]
  [mode] -> Delay7/1
  Delay7/1 -> Moe_ArMo/13
  [Dd_unshaped] -> Moe_ArMo/14
  [Kd] -> Moe_ArMo/15
  Moe_ArMo/5 -> [tau_rr]
  [tau_rr] -> Delay8/1
  Delay8/1 -> Moe_ArMo/16
  [taucX_ist] -> Moe_ArMo/17
  Moe_ArMo/13 -> [sigma_activ_list]
  Moe_ArMo/14 -> [h_inter_flag]
  [dkappa] -> LowPF18/1
  [dmin_dist] -> LowPF19/1
  [J_kappa] -> Moe_ArMo/22, Scope27/1
  [J_dist] -> Moe_ArMo/23, Scope27/2
  [min_dist] -> Moe_ArMo/19
  [kappa_ist] -> Moe_ArMo/18
  [xDEE_ist] -> Scope15/1
  [xDEE_ist_filt_ms_rads] -> Scope15/2
  [MMX_ist] -> Moe_ArMo/26
  Bus Selector/21 -> [taucQa_ist]  "<taucQa>"
  [taucQa_ist] -> Moe_ArMo/27
  Moe_ArMo/3 -> [dqa_rr]
  Triggered Subsystem/1(reaction_angle_rad) -> Moe_ArMo/59, [alpha_nf_sel]
  [rueckzug_aktiv] -> Logical Operator/1
  MatrixMultiply8/1 -> [TauQa_Nm_PDX]
  [rueckzug_aktiv] -> Edge Detector/1, MATLAB Function9/1(rueckzug_aktiv)
  Edge Detector/1 -> MATLAB Function9/2(rueckzug_aktiv_edge)
  Gain6/1 -> MATLAB Function9/3(tau_in)
  MATLAB Function9/2(tau_out) -> MATLAB Function2/1(torque_desired)
  [TauQa_Nm_RR_dq] -> MATLAB Function7/2(tau_rr)
  Bus Selector/22 -> [alpha_nf]  "<alpha_nf>"
  MATLAB Function13/1(y) -> Scope30/1, [xp_soll_KSGist_KS0ist_qa]
  Moe_ArMo/16 -> [x_ist_r]
  Moe_ArMo/15 -> [x_soll_r]
  [alpha_nf] -> Triggered Subsystem/1(In1)
  [x_soll_r] -> MATLAB Function10/1(u1)
  [x_ist_r] -> MATLAB Function10/2(u2)
  Moe_ArMo/12 -> Reshape4/1
  Reshape/1 -> [dq_all]
  [q_soll_rad] -> MATLAB Function12/2(q)
  [xEE_soll_m_rad] -> MATLAB Function12/3(x)
  [qa_soll_rad] -> MATLAB Function12/1(qa)
  Bus Selector/23 -> [q_soll_rad]  "<Q_des_rad>"
  MATLAB Function12/1(kappa_soll) -> [kappa_soll]
  MATLAB Function12/2(min_dist_soll) -> [min_dist_soll]
  [kappa_ist] -> Delay5/1
  MATLAB Function8/9(det_kappa) -> Scope14/1  "det_kappa"
  MATLAB Function8/4(dJ_kappa) -> [dJ_kappa]
  [min_dist] -> Delay6/1
  MATLAB Function8/7(J_dist) -> [J_dist]
  MATLAB Function8/3(J_kappa) -> [J_kappa]
  Delay5/1 -> MATLAB Function8/7(kappa_prev)
  MATLAB Function8/2(dkappa) -> [dkappa]
  MATLAB Function8/10(det_mindist) -> Scope14/2  "det_mindist"
  [J_hredxqa_ist] -> MATLAB Function8/4(J_hredxqa_tmp)
  [q_ist_rad] -> MATLAB Function8/2(q_tmp)
  [J_kappa] -> Delay4/1
  Delay3/1 -> MATLAB Function8/6(J_dist_prev)
  MATLAB Function8/5(min_dist) -> [min_dist]
  Delay4/1 -> MATLAB Function8/5(J_kappa_prev)
  [qa_ist_rad] -> MATLAB Function8/1(qa_tmp)
  MATLAB Function8/8(dJ_dist) -> [dJ_dist]
  [J_dist] -> Delay3/1
  [xEE_ist_m_rad] -> MATLAB Function8/3(x_tmp)
  Delay6/1 -> MATLAB Function8/8(mindist_prev)
  MATLAB Function8/6(dmindist) -> [dmin_dist]
  MATLAB Function8/1(kappa) -> [kappa_ist]
  Constant14/1 -> Logical Operator/2
  Logical Operator/1 -> Moe_ArMo/58, Triggered Subsystem/Trigger
  Bus Selector/24 -> [xp_soll]  "<xp_des>"
  Bus Selector/25 -> [dxp_soll]  "<dxp_des>"
  Bus Selector/26 -> [ddxp_soll]  "<ddxp_des>"
  [xp_soll] -> Moe_ArMo/29
  [dxp_soll] -> Moe_ArMo/30
  [ddxp_soll] -> Moe_ArMo/31
  Bus Selector/28 -> [dxp_KSGj_ist]  "<dxp_KSGj>"
  Bus Selector/27 -> [xp_KSGj_ist]  "<xp_KSGj>"
  Bus Selector/29 -> [dRxp_ist]  "<dRxp>"
  Bus Selector/30 -> [J_xpqa]  "<J_xpqa>"
  [J_xpqa] -> Moe_ArMo/37
  [xp_KSGj_ist] -> Moe_ArMo/32
  Bus Selector/31 -> [J_xpqa_KS0]  "<J_xpqa_KS0>"
  [J_xpqa_KS0] -> Moe_ArMo/38
  Bus Selector/32 -> [BP_Retr_calc_run_KSGj]  "<BP_Retr_calc_run_xp>"
  [BP_Retr_calc_run_KSGj] -> Moe_ArMo/44
  Bus Selector/33 -> [dR]  "<dR>"
  Bus Selector/34 -> [R_0Gj]  "<R_0Gj>"
  [R_0Gj] -> Moe_ArMo/35
  [xp_KSGj_ist] -> MATLAB Function13/2(data)
  Bus Selector/35 -> [dJ_xpqa]  "<dJ_xpqa>"
  Bus Selector/36 -> [dJ_xpqa_KS0]  "<dJ_xpqa_KS0>"
  Bus Selector/37 -> [dxp_KS0]  "<dxp_KS0>"
  Bus Selector/38 -> [xp_KS0]  "<xp_KS0>"
  [xp_KS0] -> Moe_ArMo/41
  Moe_ArMo/11 -> Reshape2/1
  Bus Selector/39 -> [predbody_sel]  "<predbody_sel>"
  [predbody_sel] -> Moe_ArMo/43
  [xp_KS0] -> MATLAB Function13/3(data1)
  [qa_ist_rad] -> MATLAB Function13/4(data2)
  Bus Selector/40 -> [rr_level]  "<rr_level>"
  [rr_level] -> MATLAB Function7/3(rr_level)
  [rr_level] -> Moe_ArMo/45, Scope12/1
  Bus Selector/41 -> [rueck_KS0]  "<retr_CS0>"
  [rueck_KS0] -> Scope12/2, Moe_ArMo/46
  Sum7/1 -> MATLAB Function7/1(tau_ir)
  [dqa_ist_rads] -> LowPF12/1
  [dJ_hredxqa] -> LowPF11/1
  [xDEE_ist] -> LowPF10/1
  [dkappa] -> LowPF9/1, Scope22/1
  [dmin_dist] -> Scope23/1, LowPF8/1
  [dR] -> LowPF3/1
  [dxp_KSGj_ist] -> LowPF5/1
  [dRxp_ist] -> LowPF4/1
  [dJ_xpqa_KS0] -> LowPF2/1
  [dxp_KS0] -> LowPF1/1
  [dJ_xpqa] -> LowPF/1
  [xp_soll] -> MATLAB Function13/1(u)
  Mux5/1 -> [lambda_dq]
  lambda_posxy/1 -> Gain3/1  "1"
  lambda_z/1 -> Gain5/1  "2"
  lambda_kappa/1 -> Gain8/1  "3"
  lambda_dist/1 -> Gain11/1  "4"
  lambda_xpy/1 -> Gain12/1  "5"
  lambda_xp_qa/1 -> Gain13/1  "6"
  lambda_xp/1 -> Gain14/1  "7"
  lambda_dist_ddqa/1 -> Mux21/7  "7"
  lambda_dkappa_ddqa/1 -> Mux21/6  "6"
  lambda_kappa_ddqa/1 -> Mux21/5  "5"
  lambda_dz_ddqa/1 -> Mux21/4  "4"
  lambda_z_ddqa/1 -> Mux21/3  "3"
  lambda_dposxy_ddqa/1 -> Mux21/2  "2"
  lambda_posxy_ddqa/1 -> Mux21/1  "1"
  Mux21/1 -> [lambda_ddq]
  lambda_ddist_ddqa/1 -> Mux21/8  "8"
  lambda_xp_qa_ddqa/1 -> Mux21/9  "9"
  lambda_dxp_qa_ddqa/1 -> Mux21/10  "10"
  lambda_xpy_ddqa/1 -> Mux21/11  "11"
  lambda_dxpy_ddqa/1 -> Mux21/12  "12"
  lambda_xp_ddqa/1 -> Mux21/13  "13"
  lambda_dxp_ddqa/1 -> Mux21/14  "14"
  Mux22/1 -> [lambda_tau]
  lambda_kappa_tau/1 -> Mux22/1  "1"
  lambda_dkappa_tau/1 -> Mux22/2  "2"
  lambda_dist_tau/1 -> Mux22/3  "3"
  lambda_ddist_tau/1 -> Mux22/4  "4"
  lambda_xp_qa_tau/1 -> Mux22/5  "5"
  lambda_dxp_qa_tau/1 -> Mux22/6  "6"
  lambda_xpy_tau/1 -> Mux22/7  "7"
  lambda_dxpy_tau/1 -> Mux22/8  "8"
  lambda_xp_tau/1 -> Mux22/9  "9"
  lambda_dxp_tau/1 -> Mux22/10  "10"
  [lambda_dq] -> Moe_ArMo/47
  [lambda_ddq] -> Moe_ArMo/48
  [lambda_tau] -> Moe_ArMo/49
  Gain3/1 -> Mux5/1
  Gain5/1 -> Mux5/2
  Gain8/1 -> Mux5/3
  Gain11/1 -> Mux5/4
  Gain12/1 -> Mux5/5
  Gain13/1 -> Mux5/6
  Gain14/1 -> Mux5/7
  Constant13/1 -> Gain15/1
  Constant16/1 -> Gain16/1
  Gain15/1 -> Mux23/1
  Gain16/1 -> Mux23/2
  Mux23/1 -> [pd_reglerQ]
  [pd_reglerQ] -> Moe_ArMo/50
  [rueck_KS0] -> Mux25/5  "rueck_KS0"
  [rr_level] -> Mux25/4  "rr_level"
  [kappa_soll] -> Mux26/3
  [min_dist_soll] -> Mux27/3
  [h_inter_flag] -> Mux25/3  "h_inter_flag"
  [mode] -> Mux25/1  "mode"
  [h_inter] -> Mux25/2  "h_inter"
  [min_dist] -> Mux27/4
  [dkappa] -> Mux24/1
  [dmin_dist] -> Mux24/2
  [kappa_ist] -> Mux26/4
  Mux25/1 -> Bus Creator1/6  "mode_h_rrlevel_rrrueck"
  Demux4/1 -> Mux26/1
  Demux4/2 -> Mux26/2
  Mux26/1 -> Bus Creator1/7  "kappa_lim_soll_ist"
  Mux27/1 -> Bus Creator1/8  "min_dist_lim_soll_ist"
  Mux24/1 -> Bus Creator1/9  "dkappa_dmindist"
  Demux5/2 -> Mux27/2
  Demux5/1 -> Mux27/1
  const/1 -> Sum8/2
  const1/1 -> Sum9/2
  Sum9/1 -> Mux28/4
  mindist_gain/1 -> Mux28/3, Sum9/1
  Sum8/1 -> Mux28/2
  Mux28/1 -> [kappa_mindist]
  Selector6/1 -> Demux4/1
  [kappa_mindist] -> Selector6/1
  [kappa_mindist] -> Selector7/1
  Selector7/1 -> Demux5/1
  [kappa_mindist] -> Moe_ArMo/51
  lambda_dkappa_tau_entkoppelt/1 -> Mux22/11  "11"
  lambda_dmindist_tau_entkoppelt/1 -> Mux22/12  "12"
  priority_x/1 -> Moe_ArMo/52
  [alpha_nf_sel] -> Bus Creator1/10  "alpha_nf_sel"
  [xp_soll_KSGist_KS0ist_qa] -> Bus Creator1/11  "xp_soll_KSGist_KS0ist_qa"
  Bus Selector/42 -> [kappa_traj_soll]  "<kappa_traj_des>"
  Bus Selector/43 -> [mindist_traj_soll]  "<mindist_traj_des>"
  [kappa_traj_soll] -> Delay13/1
  [mindist_traj_soll] -> Delay14/1
  activate_bp_UNB/1 -> Moe_ArMo/55
  Delay13/1 -> Moe_ArMo/56
  Delay14/1 -> Moe_ArMo/57
  kappa_lim/1 -> kappa_gain/1
  kappa_gain/1 -> Mux28/1, Sum8/1
  mindist_lim_m/1 -> mindist_gain/1
  [dJ_kappa] -> TP1_impl9/1(u_raw), Mux31/1
  [dJ_dist] -> Mux32/1, TP1_impl10/1(u_raw)
  Mux31/1 -> Scope26/1
  Mux32/1 -> Scope26/2
  MATLAB Function8/11(converged_detLimit_OPspaceLimits_check) -> Scope29/1
  Moe_ArMo/17 -> [dq_Jkappa]
  Moe_ArMo/18 -> [dq_Jdist]
  MATLAB Function10/1(y) -> [x_soll_ist_Rueck]  "x_soll_ist_r"
  status_lbound/1 -> Mux36/1
  Mux36/1 -> Moe_ArMo/53
  decimal_point_zero/1 -> Mux36/2
  decimal_point_zero1/1 -> Mux37/2
  Mux37/1 -> Moe_ArMo/54
  status_lbound1/1 -> Mux37/1
  round_decimal_point_zero/1 -> Mux36/3
  round_decimal_point_zero1/1 -> Mux37/3
  Constant1/1 -> Logical Operator1/2
  [rueckzug_aktiv] -> Logical Operator1/1
  [x_soll_ist_Rueck] -> Bus Creator1/12  "x_soll_ist_Rueck"
  Moe_ArMo/19 -> [mode_nan]
  [mode_nan] -> Bus Creator1/13  "mode_nan"
  Sum6/1 -> Sum10/1
  MatrixMultiply6/1 -> Gain17/1
  [xDDEE_soll] -> MatrixMultiply6/2
  [MMX_ist] -> MatrixMultiply6/1
  Gain17/1 -> Sum10/2
  Sum10/1 -> MatrixMultiply8/2
  Gain10/1 -> Sum2/1
  Gain4/1 -> Sum7/2
  Gain7/1 -> Sum7/1
  Sum2/1 -> Gain6/1
  Moe_ArMo/20 -> [M_kappa]
  Moe_ArMo/21 -> [M_dist]
  Bus Selector/44 -> [tauCQa_ist]  "<Cred_Qa>"
  [tauCQa_ist] -> Moe_ArMo/28
  Bus Selector/45 -> [clamp_pred]  "<clamping_predicted>"
  Bus Selector/46 -> [clampBody_pred]  "<clampingChain_predicted>"
  [clamp_pred] -> Moe_ArMo/60
  [clampBody_pred] -> Moe_ArMo/61
  clampingreaction_active/1 -> Moe_ArMo/62
  Bus Selector/47 -> [traj_qap_soll_cl]  "<traj_qap_soll_cl>"
  Bus Selector/48 -> [J_q_qa]  "<Jinv_hqx_dq_dqa>"
  Bus Selector/49 -> [dJ_q_qa]  "<dJinv_hqx_dq_dqa>"
  [q_ist_rad] -> Moe_ArMo/66
  [traj_qap_soll_cl] -> Moe_ArMo/63, Scope9/1
  [J_q_qa] -> Moe_ArMo/64
  Bus Selector/50 -> [dq]  "<QD_mod_rads>"
  [clamp_pred] -> Scope7/1
  [clampBody_pred] -> Scope7/2
  lambda_clamp_qap/1 -> Gain2/1  "8"
  Gain2/1 -> Mux5/8
  Reshape2/1 -> [ddq_all]
  Reshape4/1 -> [tau_all]
  lambda_clamp_qap_ddqa/1 -> Mux21/15  "15"
  lambda_clamp_dqap_ddqa/1 -> Mux21/16  "16"
  lambda_clamp_qap_tau/1 -> Mux22/13  "13"
  lambda_clamp_qap_tau_entkoppelt/1 -> Mux22/14  "14"
  [dq] -> LowPF16/1
  [dJ_q_qa] -> LowPF17/1
  lambda_clamp_dqa_tau/1 -> Mux22/16  "16"
  lambda_clamp_dqp_tau/1 -> Mux22/17  "17"
  lambda_clamp_dqap_tau_enkoppeln/1 -> Mux22/15  "15"
  [qap_cl] -> Bus Creator1/14  "qap_cl"
  [dqap_cl] -> Bus Creator1/15  "dqap_cl"
  LowPF16/1 -> Moe_ArMo/67
  LowPF17/1 -> Moe_ArMo/65
  LowPF/1 -> Moe_ArMo/42
  LowPF1/1 -> Moe_ArMo/40
  LowPF2/1 -> Moe_ArMo/39
  LowPF3/1 -> Moe_ArMo/36
  LowPF4/1 -> Moe_ArMo/34
  LowPF5/1 -> Moe_ArMo/33
  LowPF9/1 -> Moe_ArMo/20, Scope22/2
  LowPF8/1 -> Moe_ArMo/21, Scope23/2
  LowPF10/1 -> Moe_ArMo/10
  LowPF11/1 -> Moe_ArMo/8
  LowPF12/1 -> Moe_ArMo/4
  LowPF13/1 -> Sum3/2  "de_Qa"
  LowPF18/1 -> [dkappa_filt]
  LowPF19/1 -> [dmin_dist_filt]
  TP1_impl9/1(u_filt) -> Moe_ArMo/24, Mux31/2
  TP1_impl10/1(u_filt) -> Mux32/2, Moe_ArMo/25

== system PR_Planar_Testbench_2018/Controlpanel ==
  Bus Creator : BusCreator  Inputs=12
  Bus Creator1 : BusCreator  Inputs=5
  Compare To Zero : simulink/Logic and Bit Operations/Compare To Zero  relop===  OutDataTypeStr=boolean
  Constant : Constant  Value=0  SampleTime=-1
  Delay : Delay  DelayLength=1
  Divide : Product  Inputs=*/
  Drive_to_Homepose : Constant  Value=0  SampleTime=-1
  Drive_to_Position : Constant  Value=0  SampleTime=-1
  Drive_trajectory : Constant  Value=0  SampleTime=-1
  EMERGENCY_OFF : Constant  Value=0  SampleTime=-1
  Enable_Drive : Constant  Value=0  SampleTime=-1
  Enable_PDControl : Constant  SampleTime=-1
  GUI_started : Constant  SampleTime=-1
  MATLAB Function : MATLAB Function  TreatAsAtomicUnit=on
  Mux : Mux  Inputs=3
  Reset_RS : Constant  Value=0  SampleTime=-1
  Statusword_Rot_Drive_S1 : Constant  Value=0  SampleTime=-1
  Statusword_Rot_Drive_S2 : Constant  Value=0  SampleTime=-1
  Statusword_Rot_Drive_S3 : Constant  Value=0  SampleTime=-1
  Statusword_Trans_Drive : Constant  Value=0  SampleTime=-1
  Switch : Switch  Criteria=u2 > Threshold  SaturateOnIntegerOverflow=off  InputSameDT=off
  TP_lim_gain : Constant  SampleTime=-1
  a_max : Constant  Value=2  SampleTime=-1
  mult : Product  Inputs=**
  mult1 : Product  Inputs=**
  retr_CS0 : Constant  SampleTime=-1
  rr_level : Constant  SampleTime=-1
  t_v : Constant  SampleTime=-1
  v_max : Constant  Value=0.2  SampleTime=-1
  Statusword : Outport
  Controlpanel : Outport  Port=2
  wires:
  Statusword_Rot_Drive_S1/1 -> Bus Creator1/1, MATLAB Function/1(Statusword_S1)  "Statusword_RD1"
  Statusword_Rot_Drive_S2/1 -> Bus Creator1/2, MATLAB Function/2(Statusword_S2)  "Statusword_RD2"
  Statusword_Trans_Drive/1 -> Bus Creator1/4, MATLAB Function/4(Statusword_Trans_Drive)  "Statusword_TD"
  Statusword_Rot_Drive_S3/1 -> Bus Creator1/3, MATLAB Function/3(Statusword_S3)  "Statusword_RD3"
  Drive_to_Position/1 -> Bus Creator/2  "Drive_to_Position"
  Enable_Drive/1 -> [Enable_Drive], Bus Creator/1  "Enable_Drive"
  [Enable_Drive] -> Delay/1
  MATLAB Function/1(Statusword) -> Bus Creator1/5  "Statusword"
  Delay/1 -> Compare To Zero/1
  Compare To Zero/1 -> Switch/2
  Bus Creator1/1 -> Statusword/1  "Statusword"
  Reset_RS/1 -> Switch/1  "Reset_RS"
  Constant/1 -> Switch/3
  Enable_PDControl/1 -> Bus Creator/8  "Enable_PDControl"
  Drive_to_Homepose/1 -> Bus Creator/4  "Drive_to_Homepose"
  Drive_trajectory/1 -> Bus Creator/3  "Drive_trajectory"
  EMERGENCY_OFF/1 -> Bus Creator/5  "EMERGENCY_OFF"
  GUI_started/1 -> Bus Creator/6  "GUI_started"
  Switch/1 -> Bus Creator/7  "Reset_RS"
  rr_level/1 -> Bus Creator/9  "rr_level"
  retr_CS0/1 -> Bus Creator/10  "retr_CS0"
  Bus Creator/1 -> Controlpanel/1  "Controlpanel"
  a_max/1 -> mult1/1
  TP_lim_gain/1 -> Bus Creator/12, mult1/2, mult/2, Divide/2  "TP_gain"
  mult1/1 -> Mux/3
  v_max/1 -> mult/1
  Divide/1 -> Mux/1
  Mux/1 -> Bus Creator/11  "tv_vmax_amax"
  t_v/1 -> Divide/1
  mult/1 -> Mux/2
